simulink model "iddempr1"  (Simulink 6.3)
settings: Solver=ode45  StartTime=0.0  StopTime=500  RelTol=1e-3
libraries: simulink x1
settings Model: Creator=rsingh  LastModifiedBy=rsingh  ExtModeTrigMode=oneshot  ExtModeArmWhenConnect=off  StrictBusMsg=None
settings DataIOCC: LimitDataPoints=off
settings OptimizationCC: BooleanDataType=off
settings DebuggingCC: SolverPrmCheckMsg=none  IntegerOverflowMsg=none
settings HardwareCC: TargetUnknown=on

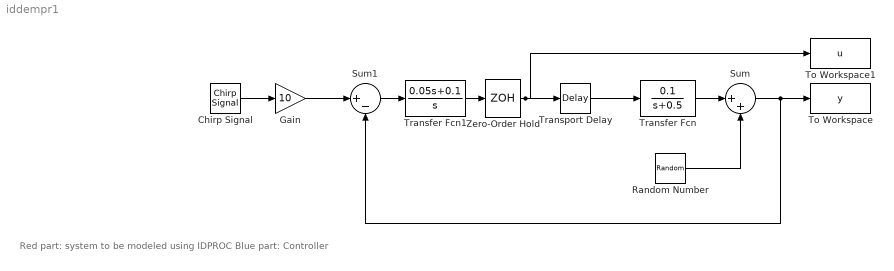
== system iddempr1 ==
  note: Red part: system to be modeled using IDPROC
      | Blue part: Controller
  Chirp Signal : simulink/Sources/Chirp Signal  f1=0.001  T=500  f2=0.2
  Gain : Gain  Gain=10  SaturateOnIntegerOverflow=on
  Random Number : RandomNumber  Variance=0.01  SampleTime=0.5
  Sum : Sum  Inputs=|++  SaturateOnIntegerOverflow=on  InputSameDT=on
  Sum1 : Sum  Inputs=|+-  SaturateOnIntegerOverflow=on  InputSameDT=on
  To Workspace : ToWorkspace  VariableName=y  SampleTime=0.5  SaveFormat=Array
  To Workspace1 : ToWorkspace  VariableName=u  SampleTime=0.5  SaveFormat=Array
  Transfer Fcn : TransferFcn  Numerator=0.1  Denominator=[1 0.5]
  Transfer Fcn1 : TransferFcn  Numerator=[0.05 0.1]  Denominator=[1 0]
  Transport Delay : TransportDelay  DelayTime=1.57
  Zero-Order Hold : ZeroOrderHold
  wires:
  Transport Delay/1 -> Transfer Fcn/1
  Transfer Fcn/1 -> Sum/1
  Random Number/1 -> Sum/2
  Sum1/1 -> Transfer Fcn1/1
  Sum/1 -> To Workspace/1, Sum1/2
  Transfer Fcn1/1 -> Zero-Order Hold/1
  Zero-Order Hold/1 -> To Workspace1/1, Transport Delay/1
  Chirp Signal/1 -> Gain/1
  Gain/1 -> Sum1/1
